simulink model "QPSK"  (R2019b)
settings: Solver=VariableStepAuto  StartTime=0.0  StopTime=10.0  MaxStep=0.0001  RelTol=1e-3
libraries: commdigbbndpm3 x2, commchan3 x1, commrandsrc3 x1
settings Model: Creator=MOSA  LastModifiedBy=Lenovo
settings DebuggingCC: SFMachineParentedDataDiag=error
settings SFSimCC: CustomCodeUndefinedFunction=UseInterfaceOnly

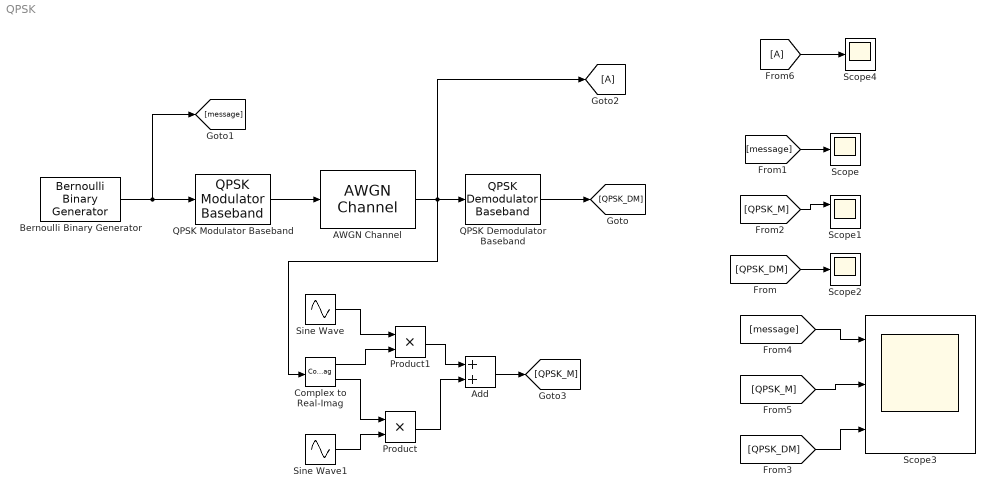
== system QPSK ==
  AWGN Channel : commchan3/AWGN Channel  InputProcessing=Columns as channels (frame based)  seed=67  noiseMode="Signal to noise ratio  (SNR)"  EbNodB=10  EsNodB=10  SNRdB=15  bitsPerSym=1  Ps=1  Tsym=1  variance=1
      settings: SourceProductName=Communications Toolbox
  Add : Sum
  Bernoulli Binary Generator : commrandsrc3/Bernoulli Binary Generator  ProbabilityOfZero=0.5  SeedSource=Parameter  Seed=67  SampleTime=0.4  SamplesPerFrame=1  OutputDataType=double  SimulateUsing=Interpreted execution
      settings: SourceProductName=Communications Toolbox
  Complex to Real-Imag : ComplexToRealImag
  Product : Product
  Product1 : Product
  QPSK Demodulator Baseband : commdigbbndpm3/QPSK Demodulator Baseband  OutType=Integer  DecType=Hard decision  VarSource=Dialog  Variance=1  Dec=Binary  Ph=pi/4  outDtype1=Inherit via internal rule  outDtype2=Inherit via internal rule  derotateFactorWordLen=16  derotateFactorDataTypeStr=Inherit: Same word length as input  derotateFactorLastDataTypeStr=Inherit: Same word length as input
      settings: SourceProductName=Communications Toolbox
  QPSK Modulator Baseband : commdigbbndpm3/QPSK Modulator Baseband  InType=Integer  Enc=Binary  Ph=pi/4  outDtype=double  outWordLen=16  outUDDataType=sfix(16)  outFracLenMode=Best precision  outFracLen=15  outDataTypeStr=double  outLastDataTypeStr=double
      settings: SourceProductName=Communications Toolbox
  Scope : Scope
  Scope1 : Scope  NumInputPorts=2
  Scope2 : Scope
  Scope3 : Scope  NumInputPorts=3
  Scope4 : Scope
  Sine Wave : Sin  Frequency=2*pi*5  SampleTime=0
  Sine Wave1 : Sin  Frequency=2*pi*5  Phase=pi/2  SampleTime=0
  wires:
  QPSK Demodulator Baseband/1 -> [QPSK_DM]
  QPSK Modulator Baseband/1 -> AWGN Channel/1
  Bernoulli Binary Generator/1 -> [message], QPSK Modulator Baseband/1
  [QPSK_M] -> Scope1/1
  [message] -> Scope/1
  [QPSK_DM] -> Scope2/1
  [QPSK_DM] -> Scope3/3
  [message] -> Scope3/1
  [QPSK_M] -> Scope3/2
  Sine Wave/1 -> Product1/1
  Complex to Real-Imag/1 -> Product1/2
  Complex to Real-Imag/2 -> Product/1
  Sine Wave1/1 -> Product/2
  Product/1 -> Add/2
  Product1/1 -> Add/1
  Add/1 -> [QPSK_M]
  AWGN Channel/1 -> [A], Complex to Real-Imag/1, QPSK Demodulator Baseband/1
  [A] -> Scope4/1
